simulink model "MMC_phase_SwitchingModel_PWMControlFrequency_20251010"  (R2024b)
settings: Solver=VariableStepAuto  StartTime=0.0  StopTime=0.35  RelTol=1e-3
values from neighbouring files (symbols this model uses):
  a = 1    [param_allsim_20250429.m]
  Ceq = 3e-3    (= 0.003)    [param_allsim_20250429.m]
  f0 = 50    [param_allsim_20250429.m]
  Fc = 1e3    (= 1000)    [param_allsim_20250429.m]
  L_ac = 100e-6    (= 0.0001)    [param_allsim_20250429.m]
  L_arm = 1e-3    (= 0.001)    [param_allsim_20250429.m]
  m = 1    [param_allsim_20250429.m]
  N = 6    [param_allsim_20250429.m]
  R = 1e-6    (= 1e-06)    [param_allsim_20250429.m]
  R_ac = 1    [param_allsim_20250429.m]
  R_arm = 1e-2    (= 0.01)    [param_allsim_20250429.m]
  VDC = 800    [param_allsim_20250429.m]
undefined symbols (not defined in the file or in its folder): C1, C_SM, L
libraries: spsSeriesRLCBranchLib x5, spsCurrentMeasurementLib x4, spsVoltageMeasurementLib x4, spsDCVoltageSourceLib x2, spsHalfBridgeMMCLib x2, spsPWMGeneratorMultilevelLib x2, spsGroundLib x1, spsTriangleGeneratorLib x1, spsMeanLib x1, spspowerguiLib x1
settings Model: Creator=ana  LastModifiedBy=ana

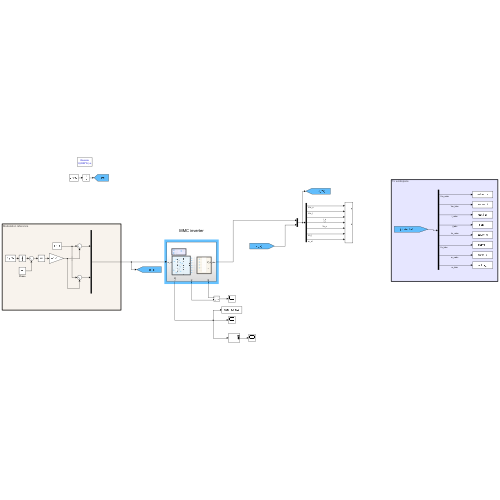
[thumbnail: Simulink's stored preview of the top-level diagram]
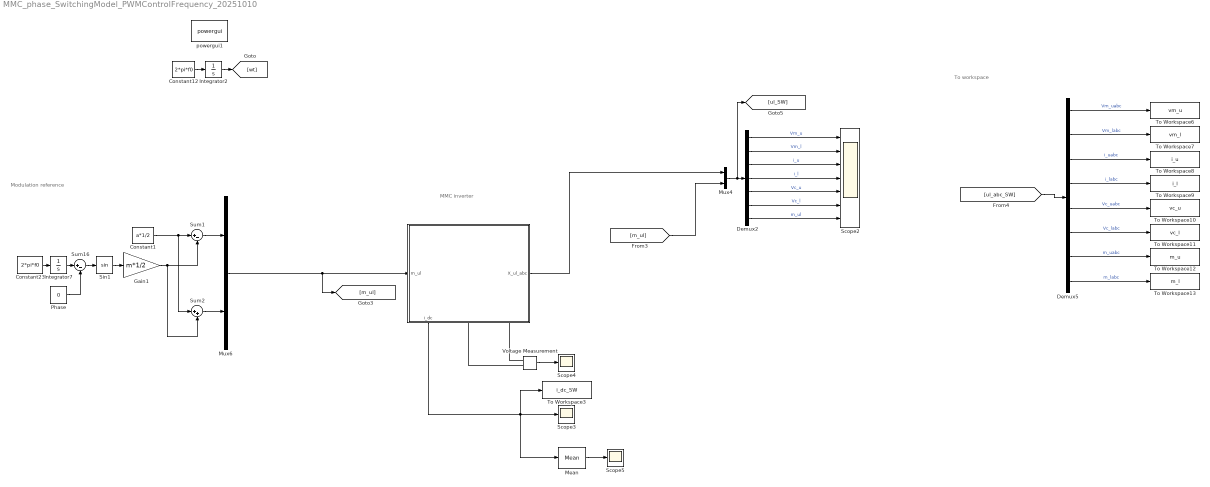
== system MMC_phase_SwitchingModel_PWMControlFrequency_20251010 ==
  note: MMC inverter
  note: To workspace
  note: Modulation reference
  " " : Subsystem
      settings: PortSchema="{\"entries\":[{\"content\":{\"sides\":[{\"content\":{\"connectorIds\":[\"In1\"]},\"type\":\"ConnectorPlacement.EquallySpacedRectSide\",\"uuid\":\"1684c177-0f69-459b-8ce9-190a6cc7c2f7\"},{\"content\":{\"connectorIds\":[\"Out1\"],\"side\":\"RIGHT\"},\"type\":\"ConnectorPlacement.EquallySpacedRectSide\",\"uuid\":\"0bff5431-30f2-45f3-9612-3e8ee114177b\"},{\"content\":{\"side\":\"TOP\"},\"type\":\"ConnectorPlacement.EquallySpacedRectSide\",\"uuid\":\"5880dbee-f5bf-4d11-b41f-6e883d19a036\"},{\"content\":{\"connectorIds\":[\"Out2\",\"RConn1\",\"RConn2\"],\"side\":\"BOTTOM\"},\"type\":\"ConnectorPlacement.EquallySpacedRectSide\",\"uuid\":\"e7f28e42-6c15-4753-aad9-7fd8153dbb2b\"}]},\"type\":\"ConnectorPlacement.EquallySpacedConnector\",\"uuid\":\"d5dc9c97-4c49-4fa9-8e0e-631ade92c721\"}],\"packageUris\":[\"http://schema.mathworks.com/mf0/Connector/R2020b\"],\"version\":\"1.0\"}"
  Constant1 : Constant  Value=a*1/2
  Constant12 : Constant  Value=2*pi*f0
  Constant23 : Constant  Value=2*pi*f0
  Demux2 : Demux  Outputs=7
  Demux5 : Demux  Outputs=8
  Gain1 : Gain  Gain=m*1/2
  Integrator2 : Integrator
  Integrator7 : Integrator
  Mean : spsMeanLib/Mean  Freq=500  Vinit=0  Ts=0
  Mux4 : Mux  Inputs=2
  Mux6 : Mux  Inputs=2
  Phase : Constant  Value=0
  Scope2 : Scope  NumInputPorts=7
  Scope3 : Scope
  Scope4 : Scope
  Scope5 : Scope
  Sin1 : Trigonometry
  Sum1 : Sum  Inputs=|+-
  Sum16 : Sum  Inputs=|+-
  Sum2 : Sum  Inputs=|++
  To Workspace10 : ToWorkspace  VariableName=vc_u  SaveFormat=Structure With Time  SampleTime=-1
      settings: MaxDataPoints=10*200000
  To Workspace11 : ToWorkspace  VariableName=vc_l  SaveFormat=Structure With Time  SampleTime=-1
      settings: MaxDataPoints=10*200000
  To Workspace12 : ToWorkspace  VariableName=m_u  SaveFormat=Structure With Time  SampleTime=-1
      settings: MaxDataPoints=10*200000
  To Workspace13 : ToWorkspace  VariableName=m_l  SaveFormat=Structure With Time  SampleTime=-1
      settings: MaxDataPoints=10*200000
  To Workspace3 : ToWorkspace  VariableName=i_dc_SW  SaveFormat=Structure With Time  SampleTime=-1
      settings: MaxDataPoints=round(10*2000*Fc/f0)
  To Workspace6 : ToWorkspace  VariableName=vm_u  SaveFormat=Structure With Time  SampleTime=-1
      settings: MaxDataPoints=10*200000
  To Workspace7 : ToWorkspace  VariableName=vm_l  SaveFormat=Structure With Time  SampleTime=-1
      settings: MaxDataPoints=10*200000
  To Workspace8 : ToWorkspace  VariableName=i_u  SaveFormat=Structure With Time  SampleTime=-1
      settings: MaxDataPoints=10*200000
  To Workspace9 : ToWorkspace  VariableName=i_l  SaveFormat=Structure With Time  SampleTime=-1
      settings: MaxDataPoints=10*200000
  Voltage Measurement : spsVoltageMeasurementLib/Voltage Measurement  PhasorSimulation=off  OutputType=Complex  PSBequivalent=0
  powergui1 : spspowerguiLib/powergui  Priority=1  SimulationMode=Discrete  SampleTime=1/(2000*Fc)  frequency=60  Iterations=50  frequencyindice=0  Pbase=100e6  ErrMax=1e-4  UnitsV=V  UnitsW=W  buscounter=0  FunctionMessages=off  echomessages=off  EnableUseOfTLC=off  CurrentSourceSwitches=off  DisableSnubberDevices=off  DisableRonSwitches=off  DisableVfSwitches=off  DisplayEquations=off  AutomaticDiscreteSolvers=off  SolverType=Backward Euler  Interpol=off  ExternalGateDelay=off  methode=off  Ts=0  x0status=blocks  SPID=off  SwTol=0  HookPort=off  NonlinearTolerance=1e-4  nMaxIteration=100  ContinueOnMaxIteration=off  RestoreLinks=warning  ResistiveCurrentMeasurement=off  Frange=[0:2:500]  Ylog=off  Xlog=on  ShowGrid=off  save=off  variable=ZData  structure=0  ZoomFFT=off  StartTime=0.0  cycles=1  DisplayStyle=1  fundamental=60  FreqAxis=off  MaxFrequency=1000  frequencyindicesteady=1  RmsSteady=1  display=off
  wires:
  " "/2(i_dc) -> To Workspace3/1, Scope3/1, Mean/1
  [m_ul] -> Mux4/2
  Constant12/1 -> Integrator2/1
  " "/1(X_ul_abc) -> Mux4/1
  Mean/1 -> Scope5/1
  Mux4/1 -> [ul_SW], Demux2/1
  Integrator2/1 -> [wt]
  Voltage Measurement/1 -> Scope4/1
  Demux2/3 -> Scope2/3  "i_u"
  Demux2/1 -> Scope2/1  "Vm_u"
  Demux2/4 -> Scope2/4  "i_l"
  Demux2/5 -> Scope2/5  "Vc_u"
  Demux2/6 -> Scope2/6  "Vc_l"
  Demux2/7 -> Scope2/7  "m_ul"
  Demux2/2 -> Scope2/2  "Vm_l"
  Demux5/6 -> To Workspace11/1  "Vc_labc"
  [ul_abc_SW] -> Demux5/1
  Demux5/4 -> To Workspace9/1  "i_labc"
  Demux5/1 -> To Workspace6/1  "Vm_uabc"
  Demux5/2 -> To Workspace7/1  "Vm_labc"
  Demux5/8 -> To Workspace13/1  "m_labc"
  Demux5/3 -> To Workspace8/1  "i_uabc"
  Demux5/5 -> To Workspace10/1  "Vc_uabc"
  Demux5/7 -> To Workspace12/1  "m_uabc"
  Constant23/1 -> Integrator7/1
  Constant1/1 -> Sum2/1, Sum1/1
  Sum2/1 -> Mux6/2
  Sin1/1 -> Gain1/1
  Sum1/1 -> Mux6/1
  Mux6/1 -> " "/1(m_ul), [m_ul]
  Gain1/1 -> Sum2/2, Sum1/2
  Integrator7/1 -> Sum16/1
  Phase/1 -> Sum16/2
  Sum16/1 -> Sin1/1
  connections:
  Voltage Measurement/LConn1 -- " "/RConn1
  Voltage Measurement/LConn2 -- " "/RConn2

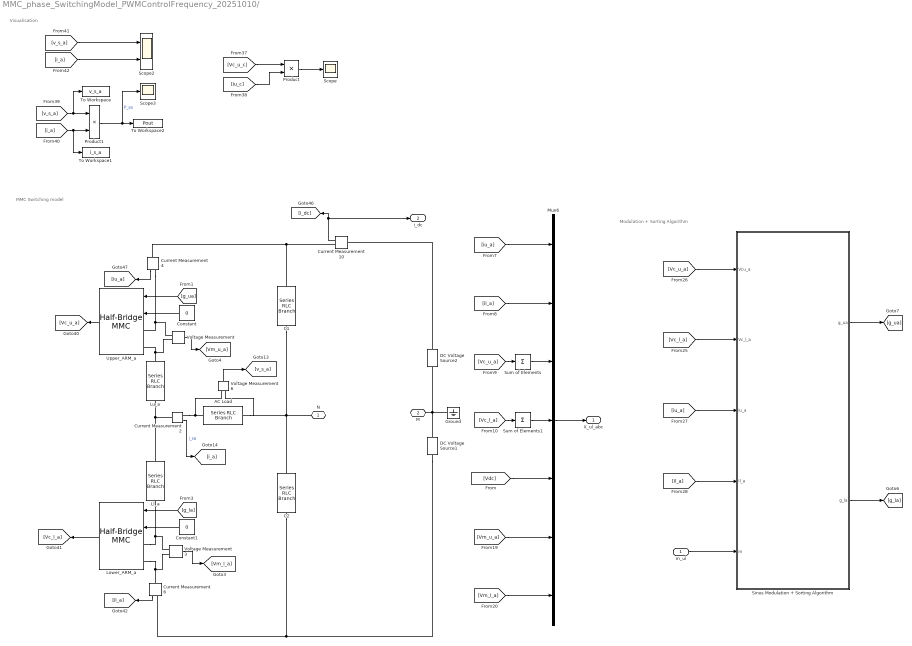
== system MMC_phase_SwitchingModel_PWMControlFrequency_20251010/  ==
  note: Visualisation
  note: Modulation + Sorting Algorithm
  note: MMC Switching model
  m_ul : Inport
  AC Load : spsSeriesRLCBranchLib/Series RLC Branch  LConnTagsString=__new0  RConnTagsString=__new0  BranchType=RL  Resistance=R_ac  Inductance=L_ac  SetiL0=off  InitialCurrent=0  Capacitance=C_SM  Setx0=off  InitialVoltage=0  Measurements=None
  C1 : spsSeriesRLCBranchLib/Series RLC Branch  LConnTagsString=__new0  RConnTagsString=__new0  BranchType=C  Resistance=R  Inductance=L  SetiL0=off  InitialCurrent=0  Capacitance=C1  Setx0=off  InitialVoltage=0  Measurements=Branch voltage and current
  C2 : spsSeriesRLCBranchLib/Series RLC Branch  LConnTagsString=__new0  RConnTagsString=__new0  BranchType=C  Resistance=R  Inductance=L  SetiL0=off  InitialCurrent=0  Capacitance=C1  Setx0=off  InitialVoltage=0  Measurements=Branch voltage and current
  Constant : Constant  Value=0
  Constant1 : Constant  Value=0
  Current Measurement{2,4,6,10} (4 alike) : spsCurrentMeasurementLib/Current Measurement  PhasorSimulation=off  OutputType=Complex  PSBequivalent=0
  DC Voltage Source1 : spsDCVoltageSourceLib/DC Voltage Source  Amplitude=VDC/2  Measurements=None
  DC Voltage Source2 : spsDCVoltageSourceLib/DC Voltage Source  Amplitude=VDC/2  Measurements=None
  Ground : spsGroundLib/Ground  LConnTagsString=a
  Ll_a : spsSeriesRLCBranchLib/Series RLC Branch  LConnTagsString=__new0  RConnTagsString=__new0  BranchType=RL  Resistance=R_arm  Inductance=L_arm  SetiL0=off  InitialCurrent=0  Capacitance=C_SM  Setx0=off  InitialVoltage=0  Measurements=None
  Lower_ARM_a : spsHalfBridgeMMCLib/Half-Bridge MMC  ModelType=Switching devices  n=N  C=Ceq*N  Vc_Initial=VDC/N  Ron=1e-4  Rs=1e6  Cs=inf  Ron_Diode=1e-3  Rs_Diode=1e6  Cs_Diode=inf  Vf_Diode=1e-3  Rs_CurrentSource=inf  Ts=10e-6
  Lu_a : spsSeriesRLCBranchLib/Series RLC Branch  LConnTagsString=__new0  RConnTagsString=__new0  BranchType=RL  Resistance=R_arm  Inductance=L_arm  SetiL0=off  InitialCurrent=0  Capacitance=C_SM  Setx0=off  InitialVoltage=0  Measurements=Branch voltage and current
  Mux6 : Mux  Inputs=7
  Product : Product
  Product1 : Product
  Scope : Scope
  Scope2 : Scope  NumInputPorts=2
  Scope3 : Scope
  Sinus Modulation + Sorting Algorithm : Subsystem
  Sum of Elements : Sum  Inputs=+
  Sum of Elements1 : Sum  Inputs=+
  To Workspace : ToWorkspace  VariableName=v_s_a  SaveFormat=Structure With Time  SampleTime=-1
  To Workspace1 : ToWorkspace  VariableName=i_s_a  SaveFormat=Structure With Time  SampleTime=-1
  To Workspace2 : ToWorkspace  VariableName=Pout  SaveFormat=Structure With Time  SampleTime=-1
  Upper_ARM_a : spsHalfBridgeMMCLib/Half-Bridge MMC  ModelType=Switching devices  n=N  C=Ceq*N  Vc_Initial=VDC/N  Ron=1e-4  Rs=1e6  Cs=inf  Ron_Diode=1e-3  Rs_Diode=1e6  Cs_Diode=inf  Vf_Diode=1e-3  Rs_CurrentSource=inf  Ts=10e-6
  Voltage Measurement : spsVoltageMeasurementLib/Voltage Measurement  PhasorSimulation=off  OutputType=Complex  PSBequivalent=0
  Voltage Measurement3 : spsVoltageMeasurementLib/Voltage Measurement  PhasorSimulation=off  OutputType=Complex  PSBequivalent=0
  Voltage Measurement6 : spsVoltageMeasurementLib/Voltage Measurement  PhasorSimulation=off  OutputType=Complex  PSBequivalent=0
  N : PMIOPort  Side=Right
  M : PMIOPort  Port=2  Side=Right
  X_ul_abc : Outport
  i_dc : Outport  Port=2
  wires:
  [iu_a] -> Mux6/1
  [il_a] -> Mux6/2
  [Vc_u_a] -> Sum of Elements/1
  [Vc_l_a] -> Sum of Elements1/1
  Mux6/1 -> X_ul_abc/1
  [Vdc] -> Mux6/5
  [Vm_u_a] -> Mux6/6
  Current Measurement6/1 -> [il_a]
  [g_ua] -> Upper_ARM_a/1
  Constant/1 -> Upper_ARM_a/2
  Current Measurement4/1 -> [iu_a]
  [g_la] -> Lower_ARM_a/1
  Lower_ARM_a/1 -> [Vc_l_a]
  Constant1/1 -> Lower_ARM_a/2
  Upper_ARM_a/1 -> [Vc_u_a]
  Sinus Modulation + Sorting Algorithm/2(g_la) -> [g_la]
  Sinus Modulation + Sorting Algorithm/1(g_ua) -> [g_ua]
  [iu_a] -> Sinus Modulation + Sorting Algorithm/3(iu_a)
  [il_a] -> Sinus Modulation + Sorting Algorithm/4(Il_a)
  [Vc_u_a] -> Sinus Modulation + Sorting Algorithm/1(Vcu_a)
  [Vc_l_a] -> Sinus Modulation + Sorting Algorithm/2(Vc_l_a)
  m_ul/1 -> Sinus Modulation + Sorting Algorithm/5(m)
  Sum of Elements/1 -> Mux6/3
  Sum of Elements1/1 -> Mux6/4
  [Vm_l_a] -> Mux6/7
  Current Measurement10/1 -> i_dc/1, [i_dc]
  [Vc_u_c] -> Product/1
  [iu_c] -> Product/2
  Product/1 -> Scope/1
  Voltage Measurement3/1 -> [Vm_l_a]
  Voltage Measurement/1 -> [Vm_u_a]
  Product1/1 -> Scope3/1, To Workspace2/1  "P_sa"
  Voltage Measurement6/1 -> [v_s_a]
  Current Measurement2/1 -> [i_a]  "i_sa"
  [v_s_a] -> To Workspace/1, Product1/1
  [i_a] -> Product1/2, To Workspace1/1
  [v_s_a] -> Scope2/1
  [i_a] -> Scope2/2
  connections:
  DC Voltage Source1/LConn1 -- C2/RConn1 -- Current Measurement6/RConn1
  DC Voltage Source1/RConn1 -- Ground/LConn1 -- M/RConn1 -- DC Voltage Source2/LConn1
  Current Measurement10/RConn1 -- C1/LConn1 -- Current Measurement4/LConn1
  Ll_a/LConn1 -- Lu_a/RConn1 -- Current Measurement2/LConn1
  Current Measurement4/RConn1 -- Upper_ARM_a/LConn1 -- Voltage Measurement/LConn1
  Lower_ARM_a/LConn2 -- Voltage Measurement3/LConn2 -- Current Measurement6/LConn1
  Lower_ARM_a/LConn1 -- Voltage Measurement3/LConn1 -- Ll_a/RConn1
  Lu_a/LConn1 -- Upper_ARM_a/LConn2 -- Voltage Measurement/LConn2
  DC Voltage Source2/RConn1 -- Current Measurement10/LConn1
  C2/LConn1 -- N/RConn1 -- Voltage Measurement6/LConn1 -- AC Load/LConn1 -- C1/RConn1
  Current Measurement2/RConn1 -- Voltage Measurement6/LConn2 -- AC Load/RConn1

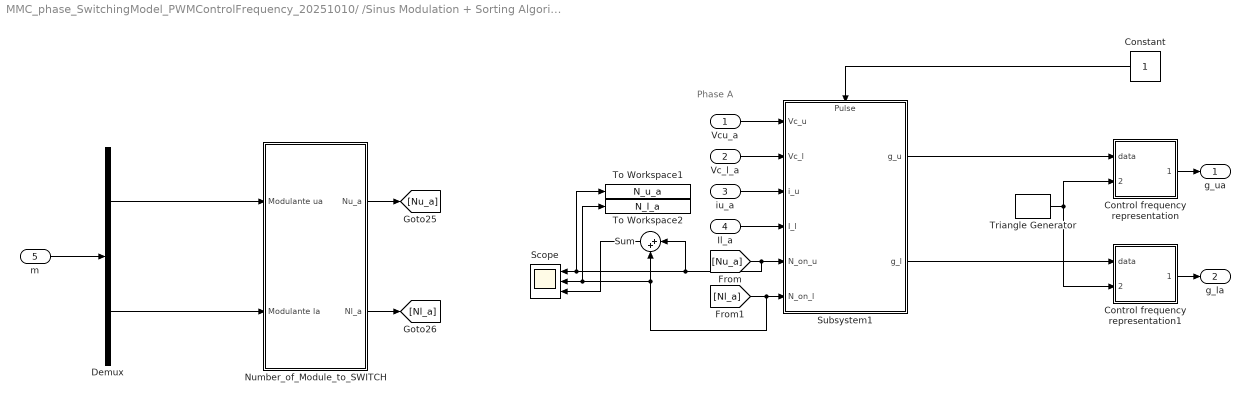
== system MMC_phase_SwitchingModel_PWMControlFrequency_20251010/ /Sinus Modulation + Sorting Algorithm ==
  note: Phase A
  Vcu_a : Inport
  Vc_l_a : Inport  Port=2
  iu_a : Inport  Port=3
  Il_a : Inport  Port=4
  m : Inport  Port=5
  Constant : Constant
  Control frequency representation : Subsystem
  Control frequency representation1 : Subsystem
  Demux : Demux  Outputs=2
  Number_of_Module_to_SWITCH : Subsystem
  Scope : Scope  NumInputPorts=3
  Subsystem1 : Subsystem
      settings: PortSchema="{\"entries\":[{\"content\":{\"sides\":[{\"content\":{\"connectorIds\":[\"In1\",\"In2\",\"In3\",\"In4\",\"In5\",\"In6\"]},\"type\":\"ConnectorPlacement.EquallySpacedRectSide\",\"uuid\":\"edb50160-a239-40a6-972c-a715a6fbe13d\"},{\"content\":{\"connectorIds\":[\"Out1\",\"Out2\"],\"side\":\"RIGHT\"},\"type\":\"ConnectorPlacement.EquallySpacedRectSide\",\"uuid\":\"50795e67-0526-4c95-8fde-c2f33aa10269\"},{\"content\":{\"connectorIds\":[\"In7\"],\"side\":\"TOP\"},\"type\":\"ConnectorPlacement.EquallySpacedRectSide\",\"uuid\":\"4b9fa748-0c00-40fa-8ad9-db170ea8506d\"}]},\"type\":\"ConnectorPlacement.EquallySpacedConnector\",\"uuid\":\"80f12ca1-3964-4a1c-b648-ca12c0c72645\"}],\"packageUris\":[\"http://schema.mathworks.com/mf0/Connector/R2020b\"],\"version\":\"1.0\"}"
  Sum : Sum  Inputs=|++
  To Workspace1 : ToWorkspace  VariableName=N_u_a  SaveFormat=Structure With Time  SampleTime=-1
  To Workspace2 : ToWorkspace  VariableName=N_l_a  SaveFormat=Structure With Time  SampleTime=-1
  Triangle Generator : spsTriangleGeneratorLib/Triangle Generator  Freq=200e3  Phase=0  Ts=0
  g_ua : Outport
  g_la : Outport  Port=2
  wires:
  Il_a/1 -> Subsystem1/4(I_l)
  Vcu_a/1 -> Subsystem1/1(Vc_u)
  Vc_l_a/1 -> Subsystem1/2(Vc_l)
  iu_a/1 -> Subsystem1/3(i_u)
  [Nu_a] -> Sum/1, To Workspace1/1, Scope/1, Subsystem1/5(N_on_u)
  [Nl_a] -> Scope/2, To Workspace2/1, Sum/2, Subsystem1/6(N_on_l)
  Number_of_Module_to_SWITCH/2(Nl_a) -> [Nl_a]
  Number_of_Module_to_SWITCH/1(Nu_a) -> [Nu_a]
  m/1 -> Demux/1
  Demux/1 -> Number_of_Module_to_SWITCH/1(Modulante ua)
  Demux/2 -> Number_of_Module_to_SWITCH/2(Modulante la)
  Sum/1 -> Scope/3
  Control frequency representation/1(Control output) -> g_ua/1
  Control frequency representation1/1(Control output) -> g_la/1
  Subsystem1/1(g_u) -> Control frequency representation/1(data)
  Subsystem1/2(g_l) -> Control frequency representation1/1(data)
  Triangle Generator/1 -> Control frequency representation1/2(carrier), Control frequency representation/2(carrier)
  Constant/1 -> Subsystem1/7(Pulse)

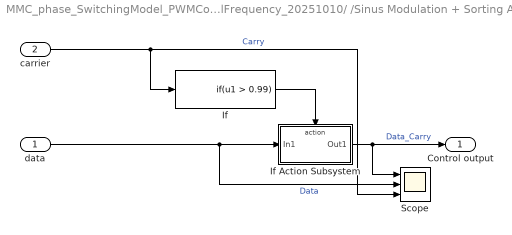
== system MMC_phase_SwitchingModel_PWMControlFrequency_20251010/ /Sinus Modulation + Sorting Algorithm/Control frequency representation ==
  data : Inport
  carrier : Inport  Port=2
  If : If  IfExpression=u1 > 0.99  ShowElse=off
  If Action Subsystem : Subsystem  TreatAsAtomicUnit=on
  Scope : Scope  NumInputPorts=3
  Control output : Outport
  wires:
  If Action Subsystem/1(Out1) -> Scope/1, Control output/1  "Data_Carry"
  data/1 -> Scope/2, If Action Subsystem/1(In1)  "Data"
  If/1 -> If Action Subsystem/Action
  carrier/1 -> If/1, Scope/3  "Carry"

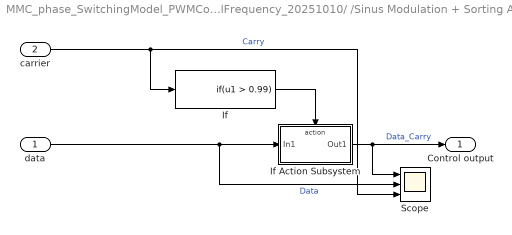
== system MMC_phase_SwitchingModel_PWMControlFrequency_20251010/ /Sinus Modulation + Sorting Algorithm/Control frequency representation1 ==
  data : Inport
  carrier : Inport  Port=2
  If : If  IfExpression=u1 > 0.99  ShowElse=off
  If Action Subsystem : Subsystem  TreatAsAtomicUnit=on
  Scope : Scope  NumInputPorts=3
  Control output : Outport
  wires:
  If Action Subsystem/1(Out1) -> Scope/1, Control output/1  "Data_Carry"
  data/1 -> Scope/2, If Action Subsystem/1(In1)  "Data"
  If/1 -> If Action Subsystem/Action
  carrier/1 -> If/1, Scope/3  "Carry"

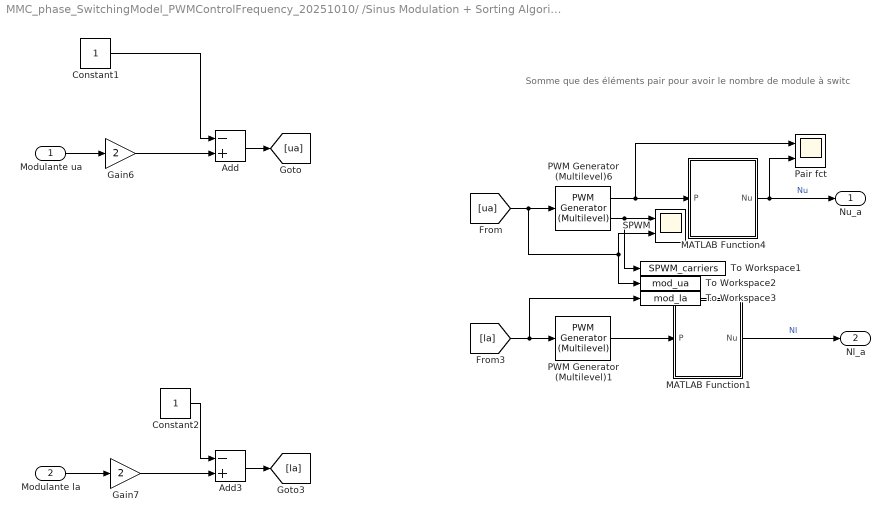
== system MMC_phase_SwitchingModel_PWMControlFrequency_20251010/ /Sinus Modulation + Sorting Algorithm/Number_of_Module_to_SWITCH ==
  note: Somme que des éléments pair pour avoir le nombre de module à switc
  Modulante ua : Inport
  Modulante la : Inport  Port=2
  Add : Sum  Inputs=-+
  Add3 : Sum  Inputs=-+
  Constant1 : Constant
  Constant2 : Constant
  Gain6 : Gain  Gain=2
  Gain7 : Gain  Gain=2
  MATLAB Function1 : MATLAB Function  TreatAsAtomicUnit=on
  MATLAB Function4 : MATLAB Function  TreatAsAtomicUnit=on
  PWM Generator (Multilevel)1 : spsPWMGeneratorMultilevelLib/PWM Generator (Multilevel)  BridgeType=Half-bridge  NumberOfBridges=N  Fc=Fc  Ts=0  ShowCarriersOutport=off
  PWM Generator (Multilevel)6 : spsPWMGeneratorMultilevelLib/PWM Generator (Multilevel)  BridgeType=Half-bridge  NumberOfBridges=N  Fc=Fc  Ts=0  ShowCarriersOutport=on
  Pair fct : Scope  NumInputPorts=2
  SPWM : Scope  NumInputPorts=2
  To Workspace1 : ToWorkspace  VariableName=SPWM_carriers  SaveFormat=Structure With Time  SampleTime=-1
  To Workspace2 : ToWorkspace  VariableName=mod_ua  SaveFormat=Structure With Time  SampleTime=-1
  To Workspace3 : ToWorkspace  VariableName=mod_la  SaveFormat=Structure With Time  SampleTime=-1
  Nu_a : Outport
  Nl_a : Outport  Port=2
  wires:
  Modulante ua/1 -> Gain6/1
  PWM Generator (Multilevel)6/1 -> Pair fct/1, MATLAB Function4/1(P)
  [ua] -> To Workspace2/1, SPWM/2, PWM Generator (Multilevel)6/1
  MATLAB Function4/1(Nu) -> Pair fct/2, Nu_a/1  "Nu"
  Modulante la/1 -> Gain7/1
  Gain6/1 -> Add/2
  Add/1 -> [ua]
  Constant1/1 -> Add/1
  Constant2/1 -> Add3/1
  Add3/1 -> [la]
  Gain7/1 -> Add3/2
  [la] -> To Workspace3/1, PWM Generator (Multilevel)1/1
  PWM Generator (Multilevel)1/1 -> MATLAB Function1/1(P)
  MATLAB Function1/1(Nu) -> Nl_a/1  "Nl"
  PWM Generator (Multilevel)6/2 -> To Workspace1/1, SPWM/1

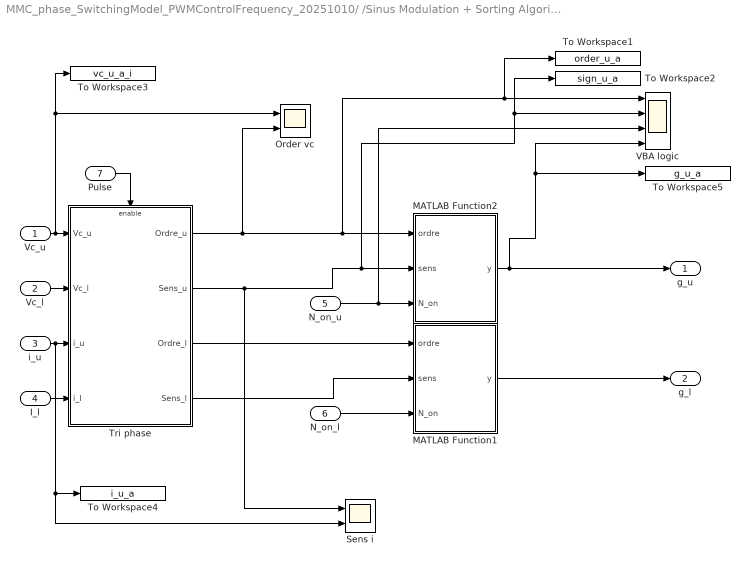
== system MMC_phase_SwitchingModel_PWMControlFrequency_20251010/ /Sinus Modulation + Sorting Algorithm/Subsystem1 ==
  Vc_u : Inport
  Vc_l : Inport  Port=2
  i_u : Inport  Port=3
  I_l : Inport  Port=4
  N_on_u : Inport  Port=5
  N_on_l : Inport  Port=6
  Pulse : Inport  Port=7
  MATLAB Function1 : MATLAB Function  TreatAsAtomicUnit=on
  MATLAB Function2 : MATLAB Function  TreatAsAtomicUnit=on
  Order vc : Scope  NumInputPorts=2
  Sens i : Scope  NumInputPorts=2
  To Workspace1 : ToWorkspace  VariableName=order_u_a  SaveFormat=Structure With Time  SampleTime=-1
  To Workspace2 : ToWorkspace  VariableName=sign_u_a  SaveFormat=Structure With Time  SampleTime=-1
  To Workspace3 : ToWorkspace  VariableName=vc_u_a_i  SaveFormat=Structure With Time  SampleTime=-1
  To Workspace4 : ToWorkspace  VariableName=i_u_a  SaveFormat=Structure With Time  SampleTime=-1
  To Workspace5 : ToWorkspace  VariableName=g_u_a  SaveFormat=Structure With Time  SampleTime=-1
  Tri phase : Subsystem
  VBA logic : Scope  NumInputPorts=4
  g_u : Outport
  g_l : Outport  Port=2
  wires:
  Vc_u/1 -> To Workspace3/1, Order vc/1, Tri phase/1(Vc_u)
  Vc_l/1 -> Tri phase/2(Vc_l)
  Tri phase/1(Ordre_u) -> To Workspace1/1, VBA logic/1, MATLAB Function2/1(ordre), Order vc/2
  N_on_u/1 -> VBA logic/3, MATLAB Function2/3(N_on)
  i_u/1 -> To Workspace4/1, Sens i/2, Tri phase/3(i_u)
  Tri phase/2(Sens_u) -> Sens i/1, VBA logic/2, To Workspace2/1, MATLAB Function2/2(sens)
  Pulse/1 -> Tri phase/Enable
  I_l/1 -> Tri phase/4(i_l)
  Tri phase/3(Ordre_l) -> MATLAB Function1/1(ordre)
  N_on_l/1 -> MATLAB Function1/3(N_on)
  Tri phase/4(Sens_l) -> MATLAB Function1/2(sens)
  MATLAB Function1/1(y) -> g_l/1
  MATLAB Function2/1(y) -> To Workspace5/1, VBA logic/4, g_u/1

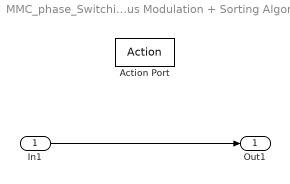
== system MMC_phase_SwitchingModel_PWMControlFrequency_20251010/ /Sinus Modulation + Sorting Algorithm/Control frequency representation/If Action Subsystem ==
  In1 : Inport
  Action Port : ActionPort
  Out1 : Outport
  wires:
  In1/1 -> Out1/1

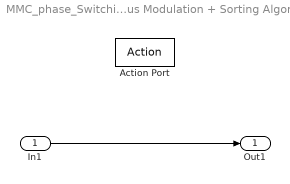
== system MMC_phase_SwitchingModel_PWMControlFrequency_20251010/ /Sinus Modulation + Sorting Algorithm/Control frequency representation1/If Action Subsystem ==
  In1 : Inport
  Action Port : ActionPort
  Out1 : Outport
  wires:
  In1/1 -> Out1/1

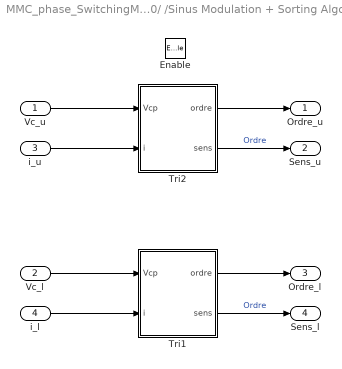
== system MMC_phase_SwitchingModel_PWMControlFrequency_20251010/ /Sinus Modulation + Sorting Algorithm/Subsystem1/Tri phase ==
  Vc_u : Inport
  Vc_l : Inport  Port=2
  i_u : Inport  Port=3
  i_l : Inport  Port=4
  Enable : EnablePort
  Tri1 : MATLAB Function  TreatAsAtomicUnit=on
  Tri2 : MATLAB Function  TreatAsAtomicUnit=on
  Ordre_u : Outport
  Sens_u : Outport  Port=2
  Ordre_l : Outport  Port=3
  Sens_l : Outport  Port=4
  wires:
  Vc_u/1 -> Tri2/1(Vcp)
  i_u/1 -> Tri2/2(i)
  Vc_l/1 -> Tri1/1(Vcp)
  i_l/1 -> Tri1/2(i)
  Tri2/1(ordre) -> Ordre_u/1
  Tri2/2(sens) -> Sens_u/1  "Ordre"
  Tri1/2(sens) -> Sens_l/1  "Ordre"
  Tri1/1(ordre) -> Ordre_l/1

== matlab function MMC_phase_SwitchingModel_PWMControlFrequency_20251010/ /Sinus Modulation + Sorting Algorithm/Number_of_Module_to_SWITCH/MATLAB Function4 ==
  data: Nu output; P input
function Nu = fcn(P)

s=0;

for k = 1:2:length(P)
    s=s+P(k);
end

Nu=s;

== matlab function MMC_phase_SwitchingModel_PWMControlFrequency_20251010/ /Sinus Modulation + Sorting Algorithm/Number_of_Module_to_SWITCH/MATLAB Function1 ==
  data: Nu output; P input
function Nu = fcn(P)

s=0;

for k = 1:2:length(P)
    s=s+P(k);
end

Nu=s;

== matlab function MMC_phase_SwitchingModel_PWMControlFrequency_20251010/ /Sinus Modulation + Sorting Algorithm/Subsystem1/Tri phase/Tri2 ==
  data: ordre output; Vcp input; i input; sens output
function [ordre,sens] = fcn(Vcp, i)

[~, ordre] = sort(Vcp);

if i > 0 
    sens = 1;
else 
    sens = 0;
end

== matlab function MMC_phase_SwitchingModel_PWMControlFrequency_20251010/ /Sinus Modulation + Sorting Algorithm/Subsystem1/Tri phase/Tri1 ==
  data: ordre output; Vcp input; i input; sens output
function [ordre,sens] = fcn(Vcp, i)

[~, ordre] = sort(Vcp);

if i > 0 
    sens = 1;
else 
    sens = 0;
end

== matlab function MMC_phase_SwitchingModel_PWMControlFrequency_20251010/ /Sinus Modulation + Sorting Algorithm/Subsystem1/MATLAB Function2 ==
  data: ordre input; y output; sens input; N_on input
function y = fcn(ordre,sens,N_on)

N_m = length(ordre);
Gp = zeros(1,2*N_m);
Ap0=ordre;

%% Sens positif (sens = 1)
if sens==1         % ON les condensateurs les moins chargés
    
    %K1 = 1 ; K2 = 0
    kp = 1:N_on;
    Gp(2*Ap0(kp))=0;
    Gp(2*Ap0(kp)-1)=1;
    
    %K1 = 0 ; K2 = 1
    kp = N_on+1:N_m;
    Gp(2*Ap0(kp))=1;
    Gp(2*Ap0(kp)-1)=0;

else            % ON les condensateurs les plus chargés
    
    %K1 = 1 ; K2 = 0
    kp = N_m:-1:N_m+1-N_on;
    Gp(2*Ap0(kp))=0;
    Gp(2*Ap0(kp)-1)=1;
    
    %K1 = 0 ; K2 = 1
    kp = N_m-N_on:-1:1;
    Gp(2*Ap0(kp))=1;
    Gp(2*Ap0(kp)-1)=0;
end
y=Gp;

== matlab function MMC_phase_SwitchingModel_PWMControlFrequency_20251010/ /Sinus Modulation + Sorting Algorithm/Subsystem1/MATLAB Function1 ==
  data: ordre input; y output; sens input; N_on input
function y = fcn(ordre,sens,N_on)

N_m = length(ordre);
Gp = zeros(1,2*N_m);
Ap0=ordre;

%% Sens positif (sens = 1)
if sens==1         % ON les condensateurs les moins chargés
    
    %K1 = 1 ; K2 = 0
    kp = 1:N_on;
    Gp(2*Ap0(kp))=0;
    Gp(2*Ap0(kp)-1)=1;
    
    %K1 = 0 ; K2 = 1
    kp = N_on+1:N_m;
    Gp(2*Ap0(kp))=1;
    Gp(2*Ap0(kp)-1)=0;

else            % ON les condensateurs les plus chargés
    
    %K1 = 1 ; K2 = 0
    kp = N_m:-1:N_m+1-N_on;
    Gp(2*Ap0(kp))=0;
    Gp(2*Ap0(kp)-1)=1;
    
    %K1 = 0 ; K2 = 1
    kp = N_m-N_on:-1:1;
    Gp(2*Ap0(kp))=1;
    Gp(2*Ap0(kp)-1)=0;
end
y=Gp;
